simulink model "Discretized_Linear_Controller_Non_Linear_Plant_STATE_SPACE_Linear_Observer"  (R2025b)
settings: Solver=VariableStepAuto  StartTime=0.0  StopTime=10  RelTol=1e-3
values from neighbouring files (symbols this model uses):
  Aobs = [p.A_lin-L*C]    [drone_controller_with_observer.m]
  Bobs = [p.B_lin L]    [drone_controller_with_observer.m]
undefined symbols (not defined in the file or in its folder): DiscIntNeverNeededParam, K, p
libraries: discretizing x1
settings Model: Creator=chako  LastModifiedBy=chako

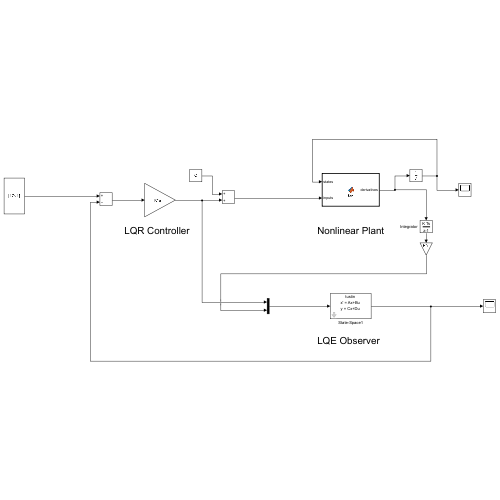
[thumbnail: Simulink's stored preview of the top-level diagram]
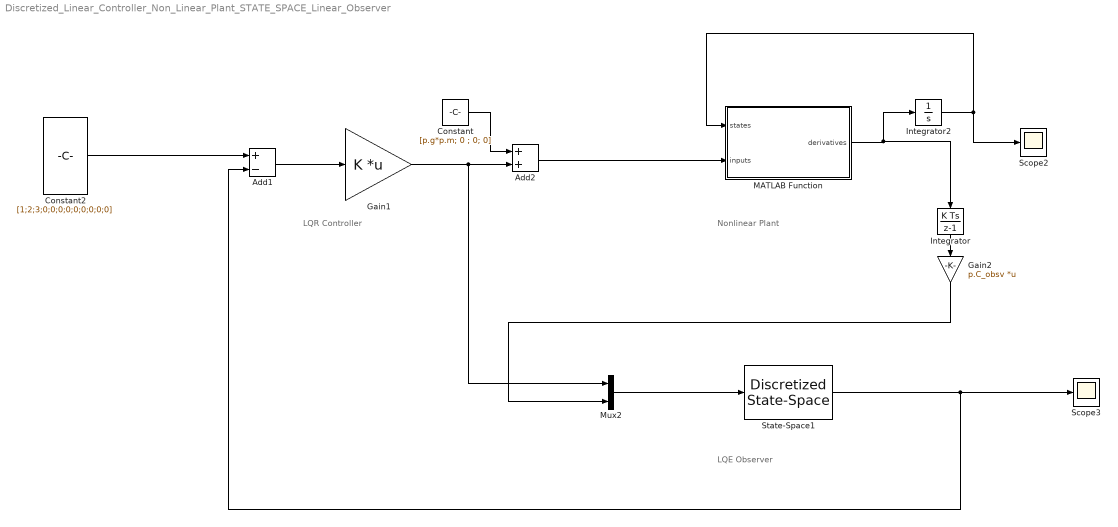
== system Discretized_Linear_Controller_Non_Linear_Plant_STATE_SPACE_Linear_Observer ==
  note: Nonlinear Plant
  note: LQR Controller
  note: LQE Observer
  Add1 : Sum  Inputs=+-
  Add2 : Sum
  Constant : Constant  Value=[p.g*p.m; 0 ; 0; 0]
  Constant2 : Constant  Value=[1;2;3;0;0;0;0;0;0;0;0;0]
  Gain1 : Gain  Gain=K  Multiplication=Matrix(K*u)
  Gain2 : Gain  Gain=p.C_obsv  Multiplication=Matrix(K*u)
  Integrator : DiscreteIntegrator  SampleTime=0.0375  ICPrevOutput=DiscIntNeverNeededParam  ICPrevScaledInput=DiscIntNeverNeededParam  mask(DiscretizedDiscreteIntegrator){}
      mask init:
      | %zoh
  Integrator2 : Integrator  InitialCondition=[0;0;0;0;0;0;0;0;0;0;0;0]
  MATLAB Function : MATLAB Function  TreatAsAtomicUnit=on
  Mux2 : Mux  Inputs=2
  Scope2 : Scope
      settings: ActiveDisplayYMinimum=-4.0288161805447356  ActiveDisplayYMaximum=14.827310955757874  DataLoggingVariableName=ScopeData2
  Scope3 : Scope
      settings: ActiveDisplayYMinimum=-15.857945347276067  ActiveDisplayYMaximum=8.2692080529825738  DataLoggingVariableName=ScopeData3
  State-Space1 : discretizing/Discretized State-Space  A=Aobs  B=Bobs  C=eye(12)  D=zeros(12, 10)  ic=0  AbsTol=auto  SampleTime=0.001  method=tustin  Wc=1
  wires:
  Gain1/1 -> Mux2/1, Add2/2
  Add2/1 -> MATLAB Function/2(inputs)
  Integrator2/1 -> MATLAB Function/1(states), Scope2/1
  Constant/1 -> Add2/1
  MATLAB Function/1(derivatives) -> Integrator/1, Integrator2/1
  Constant2/1 -> Add1/1
  Add1/1 -> Gain1/1
  State-Space1/1 -> Add1/2, Scope3/1
  Mux2/1 -> State-Space1/1
  Gain2/1 -> Mux2/2
  Integrator/1 -> Gain2/1

== matlab function Discretized_Linear_Controller_Non_Linear_Plant_STATE_SPACE_Linear_Observer/MATLAB Function ==
  data: states input size=12; derivatives output size=12; inputs input size=4; p parameter
function derivatives = fcn(states, inputs, p)

 % I is the inertia matrix
    I = [p.Ixx 0 0;
         0 p.Iyy 0;
         0 0 p.Izz];

    xi= states(1:3); % x, y, z
    xid = states(4:6); %x_prime, y_prime, z_prime
    eta = states(7:9); % roll, pitch, yaw
    etad = states(10:12); % roll_prime, pitch_prime, yaw_prime

    % Cosines of each
    c_roll = cos(eta(1));
    c_pitch = cos(eta(2));
    c_yaw = cos(eta(3));

    % Sines of each
    s_roll = sin(eta(1));
    s_pitch = sin(eta(2));
    s_yaw = sin(eta(3));


    % Derivative of xi is xid

    % Calculative derivatives of xid
    xidd = [0;0;-p.g] - (p.kD/p.m)*xid + ...
        ([s_roll*s_yaw + c_roll*s_pitch*c_yaw;
         c_roll*s_pitch*s_yaw - s_roll*c_yaw;
         c_roll*c_pitch]*inputs(1))*1/p.m; % Dividing by m here


    % Derivative of eta is etad
    % Calculative derivatives of etad


    % eta is [phi, theta, psi] = roll pitch yaw
    W = [1  0       -s_pitch;
         0  c_roll  s_roll * c_pitch;
         0 -s_roll  c_roll * c_pitch];
    % v is rpy in body frame
    
    tau_body = [inputs(2);
                inputs(3);
                inputs(4)];
    v = W * etad;
    vd = inv(I) * (tau_body + [(p.Iyy - p.Izz)*v(2)*v(3); ... 
                               (p.Izz - p.Ixx)*v(1)*v(3);
                               (p.Ixx - p.Iyy)*v(1)*v(2)]);
    Wd = [0        0                  -etad(2)*cos(-etad(2));
          0 -etad(1)*s_roll            etad(1)*c_roll*c_pitch;
          0 -etad(1)*c_roll -etad(1)*s_roll*c_pitch-etad(2)*c_roll*s_pitch];
    etadd = inv(W) * (vd - Wd*etad);
    derivatives = [xid; xidd; etad; etadd];
end
